simulink model "angle_model"  (R2023a)
settings: Solver=VariableStepAuto  StartTime=0.0  StopTime=15  RelTol=1e-3
values from neighbouring files (symbols this model uses):
  ang = 60    [script.m]
  isum = 3375    [script.m]
  Je = 0.108*10^(-6)    (= 1.08e-07)    [script.m]
  Jr = 0.016*10^(-6)    (= 1.6e-08)    [script.m]
  ke = (Un-In*R)/w    (= 0.00737661998797)    [script.m]
  km = ke    (= 0.00737661998797)    [script.m]
  Kpd = 0.855    [script.m]
  l_grab = 0.178    [script.m]
  R = 27.8    [script.m]
  Te = 0.1*Tm    (= 0.0063)    [script.m]
  Un = 12    [script.m]
libraries: checkpacklib x2, slpidlib x2
settings Model: Creator=mikha  LastModifiedBy=mikha

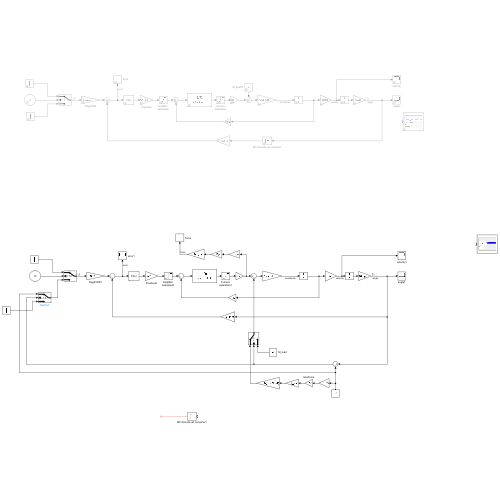
[thumbnail: Simulink's stored preview of the top-level diagram]
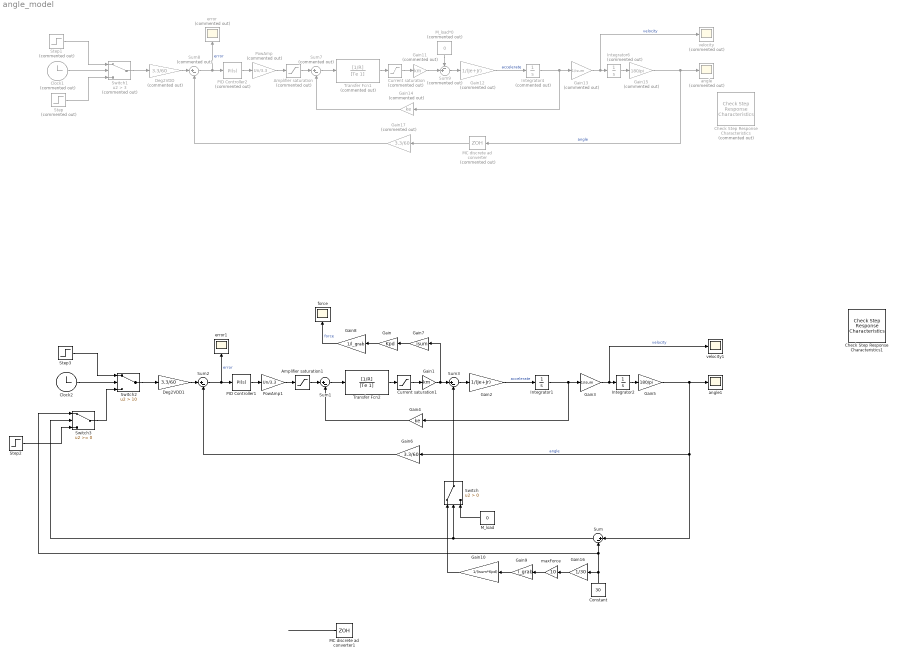
== system angle_model ==
  Amplifier saturation : Saturate  Commented=on  UpperLimit=12  LowerLimit=-12
  Amplifier saturation1 : Saturate  UpperLimit=12  LowerLimit=-12
  Check Step Response Characteristics : checkpacklib/Check Step Response  Characteristics  Commented=on  InstantiateOnLoad=on  enabled=on  stopWhenAssertionFail=off  export=off  ViewDlgPos=[513 237 510.4 389.6]  OpenViewOnLoad=off  LaunchViewOnOpen=off  TimeUnits=seconds  EnableStepResponseBound=on  InitialValue=0  FinalValue=60  StepTime=1  RiseTime=0.05  PercentRise=80  SettlingTime=0.9  PercentSettling=0  PercentOvershoot=0  PercentUndershoot=0.1
      settings: LibrarySourceBlock=|
      | sdolib/Model Verification/Check Step Response
      | Characteristics
  Check Step Response Characteristics1 : checkpacklib/Check Step Response  Characteristics  InstantiateOnLoad=on  enabled=on  stopWhenAssertionFail=off  export=off  ViewDlgPos=[513 237 510.4 389.6]  OpenViewOnLoad=off  LaunchViewOnOpen=off  TimeUnits=seconds  EnableStepResponseBound=on  InitialValue=0  FinalValue=60  StepTime=1  RiseTime=0.05  PercentRise=80  SettlingTime=0.9  PercentSettling=0  PercentOvershoot=0  PercentUndershoot=0.1
      settings: LibrarySourceBlock=|
      | sdolib/Model Verification/Check Step Response
      | Characteristics
  Clock1 : Clock  Commented=on
  Clock2 : Clock
  Constant : Constant  Value=30
  Current saturation : Saturate  Commented=on  UpperLimit=1.2  LowerLimit=-1.2
  Current saturation1 : Saturate  UpperLimit=1.2  LowerLimit=-1.2
  Deg2VDD : Gain  Commented=on  Gain=3.3/60
  Deg2VDD1 : Gain  Gain=3.3/60
  Gain : Gain  Gain=Kpd
  Gain1 : Gain  Gain=km
  Gain10 : Gain  Gain=1/(isum*Kpd)
  Gain11 : Gain  Commented=on  Gain=km
  Gain12 : Gain  Commented=on  Gain=1/(Je+Jr)
  Gain13 : Gain  Commented=on  Gain=1/isum
  Gain14 : Gain  Commented=on  Gain=ke
  Gain15 : Gain  Commented=on  Gain=180/pi
  Gain16 : Gain  Gain=1/30
  Gain17 : Gain  Commented=on  Gain=3.3/60
  Gain2 : Gain  Gain=1/(Je+Jr)
  Gain3 : Gain  Gain=1/isum
  Gain4 : Gain  Gain=ke
  Gain5 : Gain  Gain=180/pi
  Gain6 : Gain  Gain=3.3/60
  Gain7 : Gain  Gain=isum
  Gain8 : Gain  Gain=1/l_grab
  Gain9 : Gain  Gain=l_grab
  Integrator1 : Integrator
  Integrator2 : Integrator
  Integrator4 : Integrator  Commented=on
  Integrator6 : Integrator  Commented=on
  MC discrete ad converter : ZeroOrderHold  Commented=on  SampleTime=1e-4
  MC discrete ad converter1 : ZeroOrderHold  SampleTime=1e-4
  M_load : Constant  Value=0
  M_load*0 : Constant  Commented=on  Value=0
  PID Controller1 : slpidlib/PID Controller  Controller=PI  Form=Parallel  TimeDomain=Continuous-time  UseExternalTs=off  SampleTime=-1  IntegratorMethod=Forward Euler  FilterMethod=Forward Euler  ControllerParametersSource=internal  P=10.8649335654251  I=0.917356238202964  UseKiTs=off  D=0  N=100  UseFilter=on  TunerSelectOption=Transfer Function Based (PID Tuner App)  InitialConditionSource=internal  InitialConditionForIntegrator=0  InitialConditionForFilter=0  DifferentiatorICPrevScaledInput=0  ExternalReset=none  TrackingMode=off  Kt=1  LimitOutput=off  SatLimitsSource=internal  UpperSaturationLimit=inf  LowerSaturationLimit=-inf  LinearizeAsGain=on  AntiWindupMode=none  Kb=1  LimitIntegrator=off  UpperIntegratorSaturationLimit=inf  LowerIntegratorSaturationLimit=-inf  POutMin=[]  POutMax=[]  IOutMin=[]  IOutMax=[]  DOutMin=[]  DOutMax=[]  NOutMin=[]  NOutMax=[]  SumOutMin=[]  SumOutMax=[]  SaturationOutMin=[]  SaturationOutMax=[]  PParamMin=[]  PParamMax=[]  IParamMin=[]  IParamMax=[]  DParamMin=[]  DParamMax=[]  NParamMin=[]  NParamMax=[]  KbParamMin=[]  KbParamMax=[]  KtParamMin=[]  KtParamMax=[]  KbOutMin=[]  KbOutMax=[]  KtOutMin=[]  KtOutMax=[]  IntegratorOutMin=[]  IntegratorOutMax=[]  FilterOutMin=[]  FilterOutMax=[]  SumI1OutMin=[]  SumI1OutMax=[]  SumI2OutMin=[]  SumI2OutMax=[]  SumI3OutMin=[]  SumI3OutMax=[]  SumI4OutMin=[]  SumI4OutMax=[]  SumDOutMin=[]  SumDOutMax=[]  DifferentiatorOutMin=[]  DifferentiatorOutMax=[]  FilterDiffOutCoefMin=[]  FilterDiffOutCoefMax=[]  ReciprocalOutMin=[]  ReciprocalOutMax=[]  SumDenOutMin=[]  SumDenOutMax=[]  SumNumOutMin=[]  SumNumOutMax=[]  DivideOutMin=[]  DivideOutMax=[]  UdiffTsProdOutMin=[]  UdiffTsProdOutMax=[]  NTsProdOutMin=[]  NTsProdOutMax=[]  UintegralTsProdOutMin=[]  UintegralTsProdOutMax=[]  UngainTsProdOutMin=[]  UngainTsProdOutMax=[]  ClampingZeroOutDataTypeStr=Inherit: Inherit via back propagation  ClampingZeroOutMin=[]  ClampingZeroOutMax=[]  FilterDenConstantOutDataTypeStr=Inherit: Inherit via back propagation  FilterDenConstantOutMin=[]  FilterDenConstantOutMax=[]  PCopyOutDataTypeStr=Inherit: Inherit via back propagation  PCopyOutMin=[]  PCopyOutMax=[]  NCopyOutDataTypeStr=Inherit: Inherit via back propagation  NCopyOutMin=[]  NCopyOutMax=[]  IntegratorContinuousStateAttributes=''  IntegratorStateMustResolveToSignalObject=off  IntegratorRTWStateStorageClass=Auto  FilterContinuousStateAttributes=''  FilterStateMustResolveToSignalObject=off  FilterRTWStateStorageClass=Auto  ParallelPVariant=InternalParameters  IdealPVariant=Disabled  IVariant=InternalParameters  DVariant=Disabled  IntegratorVariant=Continuous  SatVariant=Disabled  AWVariant=Passthrough  PCopyVariant=Disabled  TRVariant=Disabled  FdbkBlocksVariant=Forward  IdealPFdbkVariant=Disabled  SatFdbkVariant=Disabled  DerivativeFilterVariant=Disabled  NVariant=Disabled  NCopyVariant=Disabled_SignalSpec  FilterICVariant=Disabled  IntegratorICVariant=InternalICs  ExternalResetVariant=Disabled  TRSumVariant=Passthrough  SumFdbkVariant=Disabled  SumVariant=Sum_PI  TsampFilterVariant=InternalTs  TsampNgainVariant=Passthrough  TsampIntegralVariant=Disabled_SignalSpec  ExternalSaturationOutDataTypeStr=Inherit: Same as second input
  PID Controller2 : slpidlib/PID Controller  Commented=on  Controller=PI  Form=Parallel  TimeDomain=Continuous-time  UseExternalTs=off  SampleTime=-1  IntegratorMethod=Forward Euler  FilterMethod=Forward Euler  ControllerParametersSource=internal  P=10.8649335654251  I=0.917356238202964  UseKiTs=off  D=0  N=100  UseFilter=on  TunerSelectOption=Transfer Function Based (PID Tuner App)  InitialConditionSource=internal  InitialConditionForIntegrator=0  InitialConditionForFilter=0  DifferentiatorICPrevScaledInput=0  ExternalReset=none  TrackingMode=off  Kt=1  LimitOutput=off  SatLimitsSource=internal  UpperSaturationLimit=inf  LowerSaturationLimit=-inf  LinearizeAsGain=on  AntiWindupMode=none  Kb=1  LimitIntegrator=off  UpperIntegratorSaturationLimit=inf  LowerIntegratorSaturationLimit=-inf  POutMin=[]  POutMax=[]  IOutMin=[]  IOutMax=[]  DOutMin=[]  DOutMax=[]  NOutMin=[]  NOutMax=[]  SumOutMin=[]  SumOutMax=[]  SaturationOutMin=[]  SaturationOutMax=[]  PParamMin=[]  PParamMax=[]  IParamMin=[]  IParamMax=[]  DParamMin=[]  DParamMax=[]  NParamMin=[]  NParamMax=[]  KbParamMin=[]  KbParamMax=[]  KtParamMin=[]  KtParamMax=[]  KbOutMin=[]  KbOutMax=[]  KtOutMin=[]  KtOutMax=[]  IntegratorOutMin=[]  IntegratorOutMax=[]  FilterOutMin=[]  FilterOutMax=[]  SumI1OutMin=[]  SumI1OutMax=[]  SumI2OutMin=[]  SumI2OutMax=[]  SumI3OutMin=[]  SumI3OutMax=[]  SumI4OutMin=[]  SumI4OutMax=[]  SumDOutMin=[]  SumDOutMax=[]  DifferentiatorOutMin=[]  DifferentiatorOutMax=[]  FilterDiffOutCoefMin=[]  FilterDiffOutCoefMax=[]  ReciprocalOutMin=[]  ReciprocalOutMax=[]  SumDenOutMin=[]  SumDenOutMax=[]  SumNumOutMin=[]  SumNumOutMax=[]  DivideOutMin=[]  DivideOutMax=[]  UdiffTsProdOutMin=[]  UdiffTsProdOutMax=[]  NTsProdOutMin=[]  NTsProdOutMax=[]  UintegralTsProdOutMin=[]  UintegralTsProdOutMax=[]  UngainTsProdOutMin=[]  UngainTsProdOutMax=[]  ClampingZeroOutDataTypeStr=Inherit: Inherit via back propagation  ClampingZeroOutMin=[]  ClampingZeroOutMax=[]  FilterDenConstantOutDataTypeStr=Inherit: Inherit via back propagation  FilterDenConstantOutMin=[]  FilterDenConstantOutMax=[]  PCopyOutDataTypeStr=Inherit: Inherit via back propagation  PCopyOutMin=[]  PCopyOutMax=[]  NCopyOutDataTypeStr=Inherit: Inherit via back propagation  NCopyOutMin=[]  NCopyOutMax=[]  IntegratorContinuousStateAttributes=''  IntegratorStateMustResolveToSignalObject=off  IntegratorRTWStateStorageClass=Auto  FilterContinuousStateAttributes=''  FilterStateMustResolveToSignalObject=off  FilterRTWStateStorageClass=Auto  ParallelPVariant=InternalParameters  IdealPVariant=Disabled  IVariant=InternalParameters  DVariant=Disabled  IntegratorVariant=Continuous  SatVariant=Disabled  AWVariant=Passthrough  PCopyVariant=Disabled  TRVariant=Disabled  FdbkBlocksVariant=Forward  IdealPFdbkVariant=Disabled  SatFdbkVariant=Disabled  DerivativeFilterVariant=Disabled  NVariant=Disabled  NCopyVariant=Disabled_SignalSpec  FilterICVariant=Disabled  IntegratorICVariant=InternalICs  ExternalResetVariant=Disabled  TRSumVariant=Passthrough  SumFdbkVariant=Disabled  SumVariant=Sum_PI  TsampFilterVariant=InternalTs  TsampNgainVariant=Passthrough  TsampIntegralVariant=Disabled_SignalSpec  ExternalSaturationOutDataTypeStr=Inherit: Same as second input
  PowAmp : Gain  Commented=on  Gain=Un/3.3
  PowAmp1 : Gain  Gain=Un/3.3
  Step : Step  Commented=on  Time=0  After=ang  SampleTime=0
  Step1 : Step  Commented=on  Time=3  Before=ang  After=0  SampleTime=0
  Step2 : Step  Time=0  After=ang  SampleTime=0
  Step3 : Step  Time=3  Before=ang  After=0  SampleTime=0
  Sum{,1..3} (4 alike) : Sum  Inputs=|+-
  Sum7 : Sum  Commented=on  Inputs=|+-
  Sum8 : Sum  Commented=on  Inputs=|+-
  Sum9 : Sum  Commented=on  Inputs=-+|
  Switch : Switch  Criteria=u2 > Threshold  SaturateOnIntegerOverflow=off  InputSameDT=off
  Switch1 : Switch  Commented=on  Criteria=u2 > Threshold  Threshold=3  SaturateOnIntegerOverflow=off  InputSameDT=off
  Switch2 : Switch  Criteria=u2 > Threshold  Threshold=10  SaturateOnIntegerOverflow=off  InputSameDT=off
  Switch3 : Switch  SaturateOnIntegerOverflow=off  InputSameDT=off
  Transfer Fcn1 : TransferFcn  Commented=on  Numerator=[1/R]  Denominator=[Te 1]
  Transfer Fcn2 : TransferFcn  Numerator=[1/R]  Denominator=[Te 1]
  angle : Scope  Commented=on
  angle1 : Scope
  error : Scope  Commented=on
  error1 : Scope
  force : Scope
  maxForce : Gain  Gain=10
  velocity : Scope  Commented=on
  velocity1 : Scope
  wires:
  Gain13/1 -> velocity/1, Integrator6/1  "velocity"
  Integrator4/1 -> Gain13/1, Gain14/1
  Gain14/1 -> Sum7/2
  Sum7/1 -> Transfer Fcn1/1
  Gain12/1 -> Integrator4/1  "accelerate"
  Gain15/1 -> MC discrete ad converter/1, angle/1  "angle"
  Gain11/1 -> Sum9/2
  Sum9/1 -> Gain12/1
  M_load*0/1 -> Sum9/1
  Clock1/1 -> Switch1/2
  Step1/1 -> Switch1/1
  Sum8/1 -> PID Controller2/1, error/1  "error"
  Deg2VDD/1 -> Sum8/1
  Integrator6/1 -> Gain15/1
  Gain17/1 -> Sum8/2
  Switch1/1 -> Deg2VDD/1
  Step/1 -> Switch1/3
  Transfer Fcn1/1 -> Current saturation/1
  PowAmp/1 -> Amplifier saturation/1
  PID Controller2/1 -> PowAmp/1
  Amplifier saturation/1 -> Sum7/1
  Current saturation/1 -> Gain11/1
  MC discrete ad converter/1 -> Gain17/1
  PowAmp1/1 -> Amplifier saturation1/1
  MC discrete ad converter1/1 -> ?
  Current saturation1/1 -> Gain1/1
  PID Controller1/1 -> PowAmp1/1
  Amplifier saturation1/1 -> Sum1/1
  Step3/1 -> Switch2/1
  Integrator2/1 -> Gain5/1
  Gain1/1 -> Sum3/1, Gain7/1
  Switch2/1 -> Deg2VDD1/1
  Sum2/1 -> PID Controller1/1, error1/1  "error"
  Deg2VDD1/1 -> Sum2/1
  Gain3/1 -> velocity1/1, Integrator2/1  "velocity"
  Sum3/1 -> Gain2/1
  Step2/1 -> Switch3/3
  Gain6/1 -> Sum2/2
  Clock2/1 -> Switch2/2
  Transfer Fcn2/1 -> Current saturation1/1
  Integrator1/1 -> Gain3/1, Gain4/1
  Gain5/1 -> Sum/1, Gain6/1, angle1/1  "angle"
  Sum1/1 -> Transfer Fcn2/1
  Gain2/1 -> Integrator1/1  "accelerate"
  Gain4/1 -> Sum1/2
  Gain7/1 -> Gain/1
  Gain/1 -> Gain8/1
  Gain8/1 -> force/1  "force"
  Switch/1 -> Sum3/2
  M_load/1 -> Switch/3
  Sum/1 -> Switch3/2, Switch/2
  maxForce/1 -> Gain9/1
  Constant/1 -> Switch3/1, Sum/2, Gain16/1
  Gain9/1 -> Gain10/1
  Gain10/1 -> Switch/1
  Gain16/1 -> maxForce/1
  Switch3/1 -> Switch2/3
